simulink model "Simulink_model_171120bslee"  (R2017a)
settings: Solver=ode4  StartTime=0  StopTime=1500  FixedStep=0.01  RelTol=1e-3
model workspace (MAT data in the model file):
  A = 2
  Cd = 0.35
  Jm = 0.05
  Jt = 0.00226
  Jw = 0.905
  Ki = 0.083
  Kp = 0.24
  Nf = 4
  Ni = 2.3
  Rt = 0.316
  f = 0.01
  g = 9.81
  m = 1800
  rho = 1.166
  tout = [0 1 2 3 4 5 6 7 8 9 10 11 ... (51 elements, 51x1)]
  xxx = [0 1 2 3 4 5 6 7 8 9 10 11 ... (15447 elements, 1x15447)]
  yyy = [259 259 259 259 259 259 259 259 259 259 259 259 ... (15447 elements, 1x15447)]
libraries: simulink x1
(part 2 of 2)

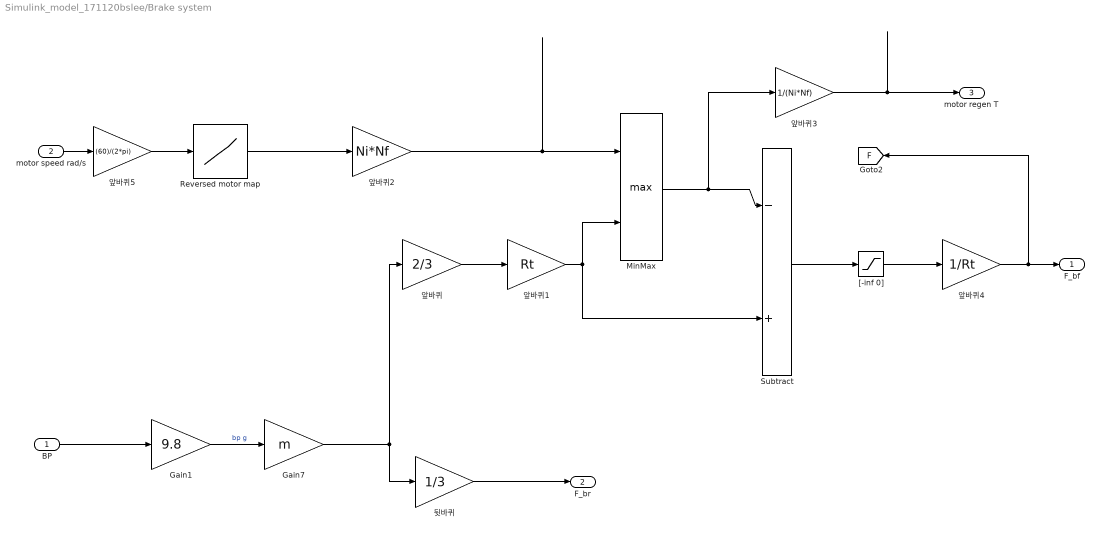
== system Simulink_model_171120bslee/Brake system ==
  BP : Inport
  motor speed rad/s : Inport  Port=2
  Gain1 : Gain  Gain=9.8
  Gain7 : Gain  Gain=m
  MinMax : MinMax  Function=max  Inputs=2
  "Reversed motor map " : Lookup_n-D  NumberOfTableDimensions=1  BreakpointsForDimension1=xxx  Table=yyy*(-1)  InternalRulePriority=Speed  RndMeth=Simplest  InputSameDT=on
  Subtract : Sum  Inputs=-+
  "[-inf 0] " : Saturate  UpperLimit=0  LowerLimit=-inf
  뒷바퀴 : Gain  Gain=1/3
  앞바퀴 : Gain  Gain=2/3
  앞바퀴1 : Gain  Gain=Rt
  앞바퀴2 : Gain  Gain=Ni*Nf
  앞바퀴3 : Gain  Gain=1/(Ni*Nf)
  앞바퀴4 : Gain  Gain=1/Rt
  앞바퀴5 : Gain  Gain=(60)/(2*pi)
  F_bf : Outport
  F_br : Outport  Port=2
  motor regen T : Outport  Port=3
  tag scope: F=global
  wires:
  BP/1 -> Gain1/1
  Gain7/1 -> 뒷바퀴/1, 앞바퀴/1
  Gain1/1 -> Gain7/1  "bp g"
  뒷바퀴/1 -> F_br/1
  앞바퀴2/1 -> MinMax/1
  motor speed rad/s/1 -> 앞바퀴5/1
  MinMax/1 -> 앞바퀴3/1, Subtract/1
  앞바퀴3/1 -> motor regen T/1
  Subtract/1 -> "[-inf 0] "/1
  "[-inf 0] "/1 -> 앞바퀴4/1
  앞바퀴4/1 -> F_bf/1, [F]
  앞바퀴/1 -> 앞바퀴1/1
  앞바퀴1/1 -> MinMax/2, Subtract/2
  앞바퀴5/1 -> "Reversed motor map "/1
  "Reversed motor map "/1 -> 앞바퀴2/1

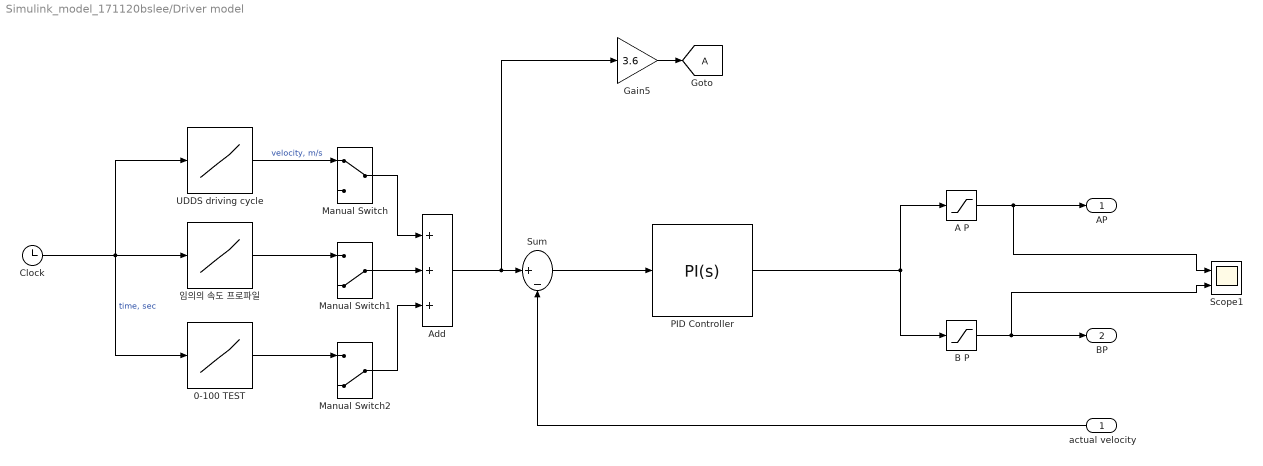
== system Simulink_model_171120bslee/Driver model ==
  actual velocity : Inport
  0-100 TEST : Lookup_n-D  NumberOfTableDimensions=1  BreakpointsForDimension1=[0 0.1 10000]  Table=[0.01 270.778 270.778]  InternalRulePriority=Speed  RndMeth=Simplest  InputSameDT=on
  A P : Saturate  UpperLimit=1  LowerLimit=0
  Add : Sum  Inputs=+++
  "B P " : Saturate  UpperLimit=0  LowerLimit=-1
  Clock : Clock
      settings: Decimation=1000
  Gain5 : Gain  Gain=3.6
  Manual Switch : ManualSwitch
  Manual Switch1 : ManualSwitch  CurrentSetting=0
  Manual Switch2 : ManualSwitch  CurrentSetting=0
  PID Controller : simulink/Continuous/PID Controller  Controller=PI  TimeDomain=Continuous-time  SampleTime=-1  IntegratorMethod=Forward Euler  FilterMethod=Forward Euler  Form=Parallel  UseFilter=on  ControllerParametersSource=internal  P=0.24  I=0.8  D=0  N=100  InitialConditionSource=internal  InitialConditionForIntegrator=0  InitialConditionForFilter=0  ExternalReset=none  LimitOutput=off  UpperSaturationLimit=inf  LowerSaturationLimit=-inf  LinearizeAsGain=on  AntiWindupMode=none  Kb=1  TrackingMode=off  Kt=1  PParamMin=[]  PParamMax=[]  IParamMin=[]  IParamMax=[]  DParamMin=[]  DParamMax=[]  NParamMin=[]  NParamMax=[]  KbParamMin=[]  KbParamMax=[]  KtParamMin=[]  KtParamMax=[]  POutMin=[]  POutMax=[]  IOutMin=[]  IOutMax=[]  DOutMin=[]  DOutMax=[]  NOutMin=[]  NOutMax=[]  KbOutMin=[]  KbOutMax=[]  KtOutMin=[]  KtOutMax=[]  IntegratorOutMin=[]  IntegratorOutMax=[]  FilterOutMin=[]  FilterOutMax=[]  SumOutMin=[]  SumOutMax=[]  SumI1OutMin=[]  SumI1OutMax=[]  SumI2OutMin=[]  SumI2OutMax=[]  SumI3OutMin=[]  SumI3OutMax=[]  SumDOutMin=[]  SumDOutMax=[]  SaturationOutMin=[]  SaturationOutMax=[]  IntegratorContinuousStateAttributes=''  IntegratorStateMustResolveToSignalObject=off  IntegratorRTWStateStorageClass=Auto  FilterContinuousStateAttributes=''  FilterStateMustResolveToSignalObject=off  FilterRTWStateStorageClass=Auto  DifferentiatorICPrevScaledInput=0  DifferentiatorOutMin=[]  DifferentiatorOutMax=[]  InitialConditionSetting=State (most efficient)
  Scope1 : Scope  NumInputPorts=2
  Sum : Sum  Inputs=|+-
  UDDS driving cycle : Lookup  InputValues=|  Table=|
      InputValues=|
      | [0	1	2	3	4	5	6	7	8	9	10	11	12	13	14	15	16	17	18	19	20	21	22	23	24	25	26	27	28	29	30	31	32	33	34	35	36	37	38	39	40	41	42	43	44	45	46	47	48	49	50	51	52	53	54	55	56	57	58	59	60	61	62	63	64	65	66	67	68	69	70	71	72	73	74	75	76	77	78	79	80	81	82	83	84	85	86	87	88	89	90	91	92	93	94	95	96	97	98	99	100	101	102	103	104	105	106	107	108	109	110	111	112	113	114	115	116	117	118	119	120	121	122	123	124	125	126	127	128	129	130	131	132	133	134	135	136	137	138	139	140	141	142	143	144	145	146	147	148	149	150	151	152	153	154	155	156	157	158	159	160	161	162	163	164	165	166	167	168	169	170	171	172	173	174	175	176	177	178	179	180	181	182	183	184	185	186	187	188	189	190	191	192	193	194	195	196	197	198	199	200	201	202	203	204	205	206	207	208	209	210	211	212	213	214	215	216	217	218	219	220	221	222	223	224	225	226	227	228	229	230	231	232	233	234	235	236	237	238	239	240	241	242	243	244	245	246	247	248	249	250	251	252	253	254	255	256	257	258	259	260	261	262	263	264	265	266	267	268	269	270	271	272	273	274	275	276	277	278	279	280	281	282	283	284	285	286	287	288	289	290	291	292	293	294	295	296	297	298	299	300	301	302	303	304	305	306	307	308	309	310	311	312	313	314	315	316	317	318	319	320	321	322	323	324	325	326	327	328	329	330	331	332	333	334	335	336	337	338	339	340	341	342	343	344	345	346	347	348	349	350	351	352	353	354	355	356	357	358	359	360	361	362	363	364	365	366	367	368	369	370	371	372	373	374	375	376	377	378	379	380	381	382	383	384	385	386	387	388	389	390	391	392	393	394	395	396	397	398	399	400	401	402	403	404	405	406	407	408	409	410	411	412	413	414	415	416	417	418	419	420	421	422	423	424	425	426	427	428	429	430	431	432	433	434	435	436	437	438	439	440	441	442	443	444	445	446	447	448	449	450	451	452	453	454	455	456	457	458	459	460	461	462	463	464	465	466	467	468	469	470	471	472	473	474	475	476	477	478	479	480	481	482	483	484	485	486	487	488	489	490	491	492	493	494	495	496	497	498	499	500	501	502	503	504	505	506	507	508	509	510	511	512	513	514	515	516	517	518	519	520	521	522	523	524	525	526	527	528	529	530	531	532	533	534	535	536	537	538	539	540	541	542	543	544	545	546	547	548	549	550	551	552	553	554	555	556	557	558	559	560	561	562	563	564	565	566	567	568	569	570	571	572	573	574	575	576	577	578	579	580	581	582	583	584	585	586	587	588	589	590	591	592	593	594	595	596	597	598	599	600	601	602	603	604	605	606	607	608	609	610	611	612	613	614	615	616	617	618	619	620	621	622	623	624	625	626	627	628	629	630	631	632	633	634	635	636	637	638	639	640	641	642	643	644	645	646	647	648	649	650	651	652	653	654	655	656	657	658	659	660	661	662	663	664	665	666	667	668	669	670	671	672	673	674	675	676	677	678	679	680	681	682	683	684	685	686	687	688	689	690	691	692	693	694	695	696	697	698	699	700	701	702	703	704	705	706	707	708	709	710	711	712	713	714	715	716	717	718	719	720	721	722	723	724	725	726	727	728	729	730	731	732	733	734	735	736	737	738	739	740	741	742	743	744	745	746	747	748	749	750	751	752	753	754	755	756	757	758	759	760	761	762	763	764	765	766	767	768	769	770	771	772	773	774	775	776	777	778	779	780	781	782	783	784	785	786	787	788	789	790	791	792	793	794	795	796	797	798	799	800	801	802	803	804	805	806	807	808	809	810	811	812	813	814	815	816	817	818	819	820	821	822	823	824	825	826	827	828	829	830	831	832	833	834	835	836	837	838	839	840	841	842	843	844	845	846	847	848	849	850	851	852	853	854	855	856	857	858	859	860	861	862	863	864	865	866	867	868	869	870	871	872	873	874	875	876	877	878	879	880	881	882	883	884	885	886	887	888	889	890	891	892	893	894	895	896	897	898	899	900	901	902	903	904	905	906	907	908	909	910	911	912	913	914	915	916	917	918	919	920	921	922	923	924	925	926	927	928	929	930	931	932	933	934	935	936	937	938	939	940	941	942	943	944	945	946	947	948	949	950	951	952	953	954	955	956	957	958	959	960	961	962	963	964	965	966	967	968	969	970	971	972	973	974	975	976	977	978	979	980	981	982	983	984	985	986	987	988	989	990	991	992	993	994	995	996	997	998	999	1000	1001	1002	1003	1004	1005	1006	1007	1008	1009	1010	1011	1012	1013	1014	1015	1016	1017	1018	1019	1020	1021	1022	1023	1024	1025	1026	1027	1028	1029	1030	1031	1032	1033	1034	1035	1036	1037	1038	1039	1040	1041	1042	1043	1044	1045	1046	1047	1048	1049	1050	1051	1052	1053	1054	1055	1056	1057	1058	1059	1060	1061	1062	1063	1064	1065	1066	1067	1068	1069	1070	1071	1072	1073	1074	1075	1076	1077	1078	1079	1080	1081	1082	1083	1084	1085	1086	1087	1088	1089	1090	1091	1092	1093	1094	1095	1096	1097	1098	1099	1100	1101	1102	1103	1104	1105	1106	1107	1108	1109	1110	1111	1112	1113	1114	1115	1116	1117	1118	1119	1120	1121	1122	1123	1124	1125	1126	1127	1128	1129	1130	1131	1132	1133	1134	1135	1136	1137	1138	1139	1140	1141	1142	1143	1144	1145	1146	1147	1148	1149	1150	1151	1152	1153	1154	1155	1156	1157	1158	1159	1160	1161	1162	1163	1164	1165	1166	1167	1168	1169	1170	1171	1172	1173	1174	1175	1176	1177	1178	1179	1180	1181	1182	1183	1184	1185	1186	1187	1188	1189	1190	1191	1192	1193	1194	1195	1196	1197	1198	1199	1200	1201	1202	1203	1204	1205	1206	1207	1208	1209	1210	1211	1212	1213	1214	1215	1216	1217	1218	1219	1220	1221	1222	1223	1224	1225	1226	1227	1228	1229	1230	1231	1232	1233	1234	1235	1236	1237	1238	1239	1240	1241	1242	1243	1244	1245	1246	1247	1248	1249	1250	1251	1252	1253	1254	1255	1256	1257	1258	1259	1260	1261	1262	1263	1264	1265	1266	1267	1268	1269	1270	1271	1272	1273	1274	1275	1276	1277	1278	1279	1280	1281	1282	1283	1284	1285	1286	1287	1288	1289	1290	1291	1292	1293	1294	1295	1296	1297	1298	1299	1300	1301	1302	1303	1304	1305	1306	1307	1308	1309	1310	1311	1312	1313	1314	1315	1316	1317	1318	1319	1320	1321	1322	1323	1324	1325	1326	1327	1328	1329	1330	1331	1332	1333	1334	1335	1336	1337	1338	1339	1340	1341	1342	1343	1344	1345	1346	1347	1348	1349	1350	1351	1352	1353	1354	1355	1356	1357	1358	1359	1360	1361	1362	1363	1364	1365	1366	1367	1368	1369
      | ]
      Table=|
      | [0
      | 0
      | 0
      | 0
      | 0
      | 0
      | 0
      | 0
      | 0
      | 0
      | 0
      | 0
      | 0
      | 0
      | 0
      | 0
      | 0
      | 0
      | 0
      | 0
      | 0
      | 1.34112000000000
      | 2.63753600000000
      | 3.84454400000000
      | 5.14096000000000
      | 6.39267200000000
      | 7.55497600000000
      | 7.73379200000000
      | 8.09142400000000
      | 9.25372800000000
      | 9.70076800000000
      | 10.0136960000000
      | 10.0584000000000
      | 9.87958400000000
      | 9.61136000000000
      | 9.34313600000000
      | 9.11961600000000
      | 8.85139200000000
      | 7.59968000000000
      | 6.66089600000000
      | 6.66089600000000
      | 6.79500800000000
      | 6.92912000000000
      | 7.15264000000000
      | 7.64438400000000
      | 8.53846400000000
      | 9.43254400000000
      | 10.1478080000000
      | 10.2372160000000
      | 10.1478080000000
      | 10.1031040000000
      | 9.52195200000000
      | 8.49376000000000
      | 7.64438400000000
      | 7.06323200000000
      | 7.06323200000000
      | 7.91260800000000
      | 8.85139200000000
      | 9.65606400000000
      | 10.3713280000000
      | 10.8183680000000
      | 10.9971840000000
      | 11.1312960000000
      | 11.1760000000000
      | 10.9971840000000
      | 10.9524800000000
      | 11.0418880000000
      | 11.0865920000000
      | 11.0418880000000
      | 10.9971840000000
      | 10.9971840000000
      | 11.2207040000000
      | 11.4442240000000
      | 11.4889280000000
      | 11.3548160000000
      | 11.1312960000000
      | 11.1760000000000
      | 11.3548160000000
      | 11.6230400000000
      | 11.6230400000000
      | 11.4889280000000
      | 11.6677440000000
      | 11.9359680000000
      | 12.2936000000000
      | 12.7853440000000
      | 13.0982720000000
      | 13.3217920000000
      | 13.4559040000000
      | 13.5900160000000
      | 13.7241280000000
      | 13.7241280000000
      | 13.6347200000000
      | 13.5900160000000
      | 13.5453120000000
      | 13.5900160000000
      | 13.7688320000000
      | 13.5900160000000
      | 13.3664960000000
      | 13.1876800000000
      | 13.3217920000000
      | 13.5453120000000
      | 13.7241280000000
      | 13.8135360000000
      | 13.8582400000000
      | 13.8135360000000
      | 13.5900160000000
      | 13.3217920000000
      | 13.3664960000000
      | 13.5006080000000
      | 13.7241280000000
      | 13.9476480000000
      | 14.2158720000000
      | 14.3946880000000
      | 14.4840960000000
      | 14.3946880000000
      | 14.1711680000000
      | 12.7853440000000
      | 11.3101120000000
      | 9.83488000000000
      | 8.35964800000000
      | 6.88441600000000
      | 5.40918400000000
      | 3.93395200000000
      | 2.45872000000000
      | 0.983488000000000
      | 0
      | 0
      | 0
      | 0
      | 0
      | 0
      | 0
      | 0
      | 0
      | 0
      | 0
      | 0
      | 0
      | 0
      | 0
      | 0
      | 0
      | 0
      | 0
      | 0
      | 0
      | 0
      | 0
      | 0
      | 0
      | 0
      | 0
      | 0
      | 0
      | 0
      | 0
      | 0
      | 0
      | 0
      | 0
      | 0
      | 0
      | 0
      | 0
      | 1.47523200000000
      | 2.95046400000000
      | 4.42569600000000
      | 5.90092800000000
      | 7.37616000000000
      | 8.85139200000000
      | 9.92428800000000
      | 10.8630720000000
      | 11.5336320000000
      | 11.8018560000000
      | 11.4889280000000
      | 11.2207040000000
      | 11.0418880000000
      | 11.1760000000000
      | 11.2654080000000
      | 11.3548160000000
      | 11.5336320000000
      | 12.1594880000000
      | 11.8465600000000
      | 10.7289600000000
      | 10.1478080000000
      | 8.67257600000000
      | 7.91260800000000
      | 7.68908800000000
      | 8.09142400000000
      | 8.31494400000000
      | 8.94080000000000
      | 9.92428800000000
      | 10.9524800000000
      | 12.2041920000000
      | 13.6347200000000
      | 14.9758400000000
      | 16.1828480000000
      | 16.6745920000000
      | 17.5686720000000
      | 18.1051200000000
      | 18.8203840000000
      | 19.4462400000000
      | 20.1615040000000
      | 20.5638400000000
      | 20.9214720000000
      | 21.2344000000000
      | 21.2344000000000
      | 21.1449920000000
      | 21.1002880000000
      | 21.0108800000000
      | 21.0108800000000
      | 21.0108800000000
      | 21.0108800000000
      | 21.0108800000000
      | 21.1002880000000
      | 21.1896960000000
      | 21.4132160000000
      | 21.6814400000000
      | 21.9496640000000
      | 22.1284800000000
      | 22.3520000000000
      | 22.6202240000000
      | 22.7990400000000
      | 23.0225600000000
      | 23.3354880000000
      | 23.7825280000000
      | 24.1848640000000
      | 24.4083840000000
      | 24.5424960000000
      | 24.5872000000000
      | 24.5424960000000
      | 24.4083840000000
      | 24.4083840000000
      | 24.4977920000000
      | 24.6319040000000
      | 24.8107200000000
      | 24.9001280000000
      | 25.0789440000000
      | 25.1683520000000
      | 25.3024640000000
      | 25.3471680000000
      | 25.3471680000000
      | 25.2577600000000
      | 25.2577600000000
      | 25.2577600000000
      | 25.2577600000000
      | 25.2577600000000
      | 25.2577600000000
      | 25.2130560000000
      | 25.0789440000000
      | 24.9448320000000
      | 24.6319040000000
      | 24.4083840000000
      | 24.2295680000000
      | 24.1401600000000
      | 24.0060480000000
      | 23.9613440000000
      | 24.0954560000000
      | 24.1401600000000
      | 24.1848640000000
      | 24.1848640000000
      | 24.0507520000000
      | 23.8719360000000
      | 23.6931200000000
      | 23.5143040000000
      | 23.2907840000000
      | 23.4248960000000
      | 23.2460800000000
      | 23.2013760000000
      | 23.1119680000000
      | 23.0225600000000
      | 23.0672640000000
      | 23.1566720000000
      | 23.2907840000000
      | 23.4696000000000
      | 23.6931200000000
      | 23.9166400000000
      | 24.1401600000000
      | 24.5424960000000
      | 24.7660160000000
      | 24.8554240000000
      | 25.0342400000000
      | 25.0342400000000
      | 24.9448320000000
      | 24.6766080000000
      | 24.3636800000000
      | 23.9613440000000
      | 23.4696000000000
      | 23.0225600000000
      | 23.0225600000000
      | 23.0225600000000
      | 22.8437440000000
      | 22.3967040000000
      | 22.3520000000000
      | 22.3967040000000
      | 22.3520000000000
      | 22.1731840000000
      | 22.1284800000000
      | 22.1284800000000
      | 22.1284800000000
      | 21.9496640000000
      | 21.7261440000000
      | 21.5026240000000
      | 21.1002880000000
      | 20.6085440000000
      | 20.1168000000000
      | 19.5803520000000
      | 19.0439040000000
      | 18.5521600000000
      | 18.0157120000000
      | 17.2110400000000
      | 16.5404800000000
      | 15.7358080000000
      | 15.1099520000000
      | 14.5288000000000
      | 14.0817600000000
      | 13.6794240000000
      | 13.6347200000000
      | 13.4112000000000
      | 12.9641600000000
      | 12.2936000000000
      | 11.0865920000000
      | 9.61136000000000
      | 8.98550400000000
      | 8.53846400000000
      | 8.27024000000000
      | 7.59968000000000
      | 6.92912000000000
      | 5.58800000000000
      | 4.82803200000000
      | 3.57632000000000
      | 2.10108800000000
      | 0.625856000000000
      | 0
      | 0
      | 0
      | 0
      | 0
      | 0
      | 0
      | 0
      | 0
      | 0
      | 0
      | 0
      | 0
      | 0
      | 0.447040000000000
      | 1.92227200000000
      | 3.39750400000000
      | 4.87273600000000
      | 6.34796800000000
      | 7.73379200000000
      | 8.94080000000000
      | 10.0584000000000
      | 10.5948480000000
      | 11.2654080000000
      | 11.8912640000000
      | 12.5618240000000
      | 13.4112000000000
      | 13.7688320000000
      | 14.1264640000000
      | 14.3499840000000
      | 14.6629120000000
      | 15.0205440000000
      | 15.4228800000000
      | 15.4675840000000
      | 15.6016960000000
      | 15.5569920000000
      | 15.4228800000000
      | 15.5122880000000
      | 15.8699200000000
      | 16.0934400000000
      | 16.0934400000000
      | 16.0934400000000
      | 16.0934400000000
      | 16.0934400000000
      | 16.0934400000000
      | 16.1381440000000
      | 16.2722560000000
      | 16.3169600000000
      | 16.2722560000000
      | 16.0934400000000
      | 15.6911040000000
      | 15.2440640000000
      | 14.9758400000000
      | 14.0370560000000
      | 12.9641600000000
      | 11.4889280000000
      | 10.2819200000000
      | 9.07491200000000
      | 7.82320000000000
      | 6.48208000000000
      | 5.36448000000000
      | 3.88924800000000
      | 2.41401600000000
      | 0.938784000000000
      | 0
      | 0
      | 0
      | 0
      | 0
      | 0
      | 1.16230400000000
      | 2.63753600000000
      | 4.11276800000000
      | 5.58800000000000
      | 7.06323200000000
      | 8.53846400000000
      | 10.0136960000000
      | 11.1760000000000
      | 11.4442240000000
      | 12.2936000000000
      | 12.9641600000000
      | 13.4112000000000
      | 13.4559040000000
      | 13.4112000000000
      | 13.2770880000000
      | 13.0982720000000
      | 12.8747520000000
      | 12.5171200000000
      | 11.1760000000000
      | 9.70076800000000
      | 8.22553600000000
      | 6.75030400000000
      | 5.27507200000000
      | 3.79984000000000
      | 2.32460800000000
      | 0.849376000000000
      | 0
      | 0
      | 0
      | 0
      | 0
      | 0
      | 0
      | 0
      | 0
      | 0
      | 0
      | 0
      | 0
      | 0
      | 0
      | 0
      | 0
      | 0
      | 0
      | 1.47523200000000
      | 2.95046400000000
      | 4.42569600000000
      | 5.90092800000000
      | 7.37616000000000
      | 8.85139200000000
      | 10.3266240000000
      | 11.8018560000000
      | 12.4277120000000
      | 13.0088640000000
      | 14.0817600000000
      | 14.7523200000000
      | 15.0205440000000
      | 15.5569920000000
      | 15.6911040000000
      | 15.9146240000000
      | 16.1381440000000
      | 16.0934400000000
      | 16.1381440000000
      | 16.1828480000000
      | 16.0934400000000
      | 15.9593280000000
      | 16.0934400000000
      | 16.0934400000000
      | 15.9146240000000
      | 15.8699200000000
      | 15.8252160000000
      | 15.7358080000000
      | 15.7358080000000
      | 15.7358080000000
      | 15.7358080000000
      | 15.7358080000000
      | 15.7358080000000
      | 15.6464000000000
      | 15.6911040000000
      | 15.7358080000000
      | 15.8699200000000
      | 15.7358080000000
      | 15.6464000000000
      | 15.6464000000000
      | 15.6464000000000
      | 15.5569920000000
      | 15.4675840000000
      | 15.4228800000000
      | 14.9758400000000
      | 14.3052800000000
      | 13.4559040000000
      | 12.5171200000000
      | 11.3995200000000
      | 10.0584000000000
      | 8.85139200000000
      | 7.37616000000000
      | 5.90092800000000
      | 4.60451200000000
      | 3.21868800000000
      | 1.78816000000000
      | 0.447040000000000
      | 0
      | 0
      | 0
      | 0
      | 0
      | 0
      | 0.536448000000000
      | 1.56464000000000
      | 2.45872000000000
      | 2.90576000000000
      | 3.79984000000000
      | 4.29158400000000
      | 4.69392000000000
      | 5.31977600000000
      | 6.25856000000000
      | 7.15264000000000
      | 7.91260800000000
      | 8.49376000000000
      | 8.98550400000000
      | 9.38784000000000
      | 9.83488000000000
      | 10.2819200000000
      | 10.6395520000000
      | 10.9524800000000
      | 11.1312960000000
      | 11.1760000000000
      | 11.1760000000000
      | 11.1760000000000
      | 11.1760000000000
      | 11.1760000000000
      | 11.1760000000000
      | 11.4442240000000
      | 11.5336320000000
      | 11.6230400000000
      | 11.4442240000000
      | 11.2654080000000
      | 11.1760000000000
      | 11.1760000000000
      | 11.1760000000000
      | 10.9077760000000
      | 10.3266240000000
      | 8.85139200000000
      | 7.37616000000000
      | 5.90092800000000
      | 4.42569600000000
      | 2.95046400000000
      | 1.47523200000000
      | 0
      | 0
      | 0
      | 0
      | 0
      | 0
      | 0
      | 0
      | 0
      | 0
      | 0
      | 0
      | 0
      | 0
      | 0
      | 0
      | 0
      | 1.47523200000000
      | 2.95046400000000
      | 4.42569600000000
      | 5.81152000000000
      | 6.52678400000000
      | 7.15264000000000
      | 7.59968000000000
      | 7.59968000000000
      | 7.59968000000000
      | 7.82320000000000
      | 7.91260800000000
      | 7.91260800000000
      | 7.82320000000000
      | 7.59968000000000
      | 7.55497600000000
      | 7.42086400000000
      | 7.59968000000000
      | 7.64438400000000
      | 7.59968000000000
      | 7.42086400000000
      | 7.37616000000000
      | 7.37616000000000
      | 7.42086400000000
      | 7.59968000000000
      | 7.86790400000000
      | 8.27024000000000
      | 8.58316800000000
      | 9.03020800000000
      | 9.38784000000000
      | 9.43254400000000
      | 9.47724800000000
      | 9.65606400000000
      | 9.83488000000000
      | 10.0136960000000
      | 10.0584000000000
      | 10.0584000000000
      | 10.0584000000000
      | 10.1478080000000
      | 10.5948480000000
      | 11.2207040000000
      | 11.6230400000000
      | 11.8465600000000
      | 12.0700800000000
      | 11.6677440000000
      | 10.1925120000000
      | 8.71728000000000
      | 7.24204800000000
      | 5.76681600000000
      | 4.29158400000000
      | 2.81635200000000
      | 1.34112000000000
      | 0
      | 0
      | 0
      | 0
      | 0
      | 0
      | 0
      | 0
      | 0
      | 0
      | 0
      | 0
      | 0
      | 0
      | 0
      | 0
      | 0
      | 0
      | 0
      | 0
      | 0
      | 0
      | 0
      | 0
      | 0
      | 0
      | 0.894080000000000
      | 2.01168000000000
      | 3.48691200000000
      | 4.55980800000000
      | 5.58800000000000
      | 6.25856000000000
      | 6.83971200000000
      | 7.82320000000000
      | 8.76198400000000
      | 9.38784000000000
      | 9.92428800000000
      | 10.4160320000000
      | 10.9524800000000
      | 11.3101120000000
      | 11.4442240000000
      | 11.6230400000000
      | 11.6677440000000
      | 11.7124480000000
      | 11.7124480000000
      | 11.8018560000000
      | 11.8465600000000
      | 11.8465600000000
      | 11.6230400000000
      | 11.3995200000000
      | 10.5501440000000
      | 9.56665600000000
      | 8.27024000000000
      | 7.33145600000000
      | 6.48208000000000
      | 5.18566400000000
      | 3.88924800000000
      | 2.59283200000000
      | 1.56464000000000
      | 0.894080000000000
      | 0
      | 0
      | 0
      | 0
      | 0
      | 0
      | 0
      | 0
      | 0
      | 0
      | 0
      | 0
      | 0
      | 0
      | 0.625856000000000
      | 1.47523200000000
      | 1.96697600000000
      | 2.90576000000000
      | 4.11276800000000
      | 5.05155200000000
      | 6.03504000000000
      | 6.52678400000000
      | 7.33145600000000
      | 7.46556800000000
      | 7.37616000000000
      | 7.37616000000000
      | 8.13612800000000
      | 8.58316800000000
      | 8.98550400000000
      | 9.61136000000000
      | 10.0584000000000
      | 10.0584000000000
      | 9.87958400000000
      | 10.1478080000000
      | 10.4160320000000
      | 10.5054400000000
      | 10.0584000000000
      | 9.65606400000000
      | 9.16432000000000
      | 8.04672000000000
      | 6.70560000000000
      | 5.36448000000000
      | 4.02336000000000
      | 2.77164800000000
      | 2.01168000000000
      | 1.34112000000000
      | 0.938784000000000
      | 0.223520000000000
      | 0.223520000000000
      | 1.43052800000000
      | 2.90576000000000
      | 4.29158400000000
      | 5.58800000000000
      | 6.25856000000000
      | 7.15264000000000
      | 8.04672000000000
      | 8.76198400000000
      | 9.61136000000000
      | 10.3266240000000
      | 10.9524800000000
      | 11.3995200000000
      | 11.8465600000000
      | 12.1147840000000
      | 12.3383040000000
      | 12.4724160000000
      | 12.6512320000000
      | 12.7853440000000
      | 12.7853440000000
      | 12.6512320000000
      | 12.6065280000000
      | 12.5171200000000
      | 12.2936000000000
      | 11.9806720000000
      | 11.3995200000000
      | 10.5054400000000
      | 9.61136000000000
      | 8.49376000000000
      | 7.37616000000000
      | 6.66089600000000
      | 5.58800000000000
      | 4.20217600000000
      | 2.77164800000000
      | 1.34112000000000
      | 0.670560000000000
      | 0.670560000000000
      | 0.223520000000000
      | 0
      | 1.34112000000000
      | 2.81635200000000
      | 4.29158400000000
      | 5.76681600000000
      | 7.06323200000000
      | 7.82320000000000
      | 8.22553600000000
      | 8.71728000000000
      | 9.25372800000000
      | 9.83488000000000
      | 10.3713280000000
      | 11.1760000000000
      | 11.8465600000000
      | 12.2936000000000
      | 12.5171200000000
      | 12.6512320000000
      | 12.9194560000000
      | 12.9194560000000
      | 12.9194560000000
      | 12.8747520000000
      | 12.7406400000000
      | 12.6512320000000
      | 12.6512320000000
      | 12.6512320000000
      | 12.6065280000000
      | 12.3383040000000
      | 12.2936000000000
      | 12.2936000000000
      | 12.2936000000000
      | 12.2936000000000
      | 12.2936000000000
      | 12.2936000000000
      | 12.3383040000000
      | 12.5171200000000
      | 12.7406400000000
      | 13.4112000000000
      | 13.8582400000000
      | 14.3052800000000
      | 14.7523200000000
      | 14.7523200000000
      | 15.0205440000000
      | 15.1993600000000
      | 15.3334720000000
      | 15.2887680000000
      | 15.1993600000000
      | 15.1993600000000
      | 15.1546560000000
      | 15.0205440000000
      | 14.7970240000000
      | 14.7523200000000
      | 14.5288000000000
      | 14.3052800000000
      | 14.2605760000000
      | 14.1264640000000
      | 14.0817600000000
      | 13.6794240000000
      | 13.4112000000000
      | 13.3664960000000
      | 13.3664960000000
      | 13.3664960000000
      | 13.3664960000000
      | 13.2323840000000
      | 13.1876800000000
      | 13.1876800000000
      | 13.0982720000000
      | 12.9194560000000
      | 12.6065280000000
      | 12.3830080000000
      | 12.0700800000000
      | 11.3995200000000
      | 10.5948480000000
      | 9.83488000000000
      | 9.16432000000000
      | 8.58316800000000
      | 8.58316800000000
      | 8.98550400000000
      | 9.34313600000000
      | 9.56665600000000
      | 9.83488000000000
      | 10.1031040000000
      | 10.3713280000000
      | 10.7289600000000
      | 11.1760000000000
      | 11.6230400000000
      | 11.8912640000000
      | 11.8912640000000
      | 11.9806720000000
      | 12.0700800000000
      | 12.1594880000000
      | 12.4277120000000
      | 12.5618240000000
      | 12.8747520000000
      | 12.9194560000000
      | 12.9641600000000
      | 13.0088640000000
      | 12.9641600000000
      | 12.5618240000000
      | 12.2936000000000
      | 12.0700800000000
      | 11.5336320000000
      | 11.1760000000000
      | 10.9524800000000
      | 11.0865920000000
      | 11.2207040000000
      | 11.3995200000000
      | 11.4889280000000
      | 11.7124480000000
      | 12.0253760000000
      | 12.2936000000000
      | 12.4277120000000
      | 12.6959360000000
      | 12.9641600000000
      | 13.0535680000000
      | 13.0088640000000
      | 12.9641600000000
      | 12.9194560000000
      | 12.7406400000000
      | 12.5618240000000
      | 12.5171200000000
      | 12.5171200000000
      | 12.3383040000000
      | 12.1594880000000
      | 11.8912640000000
      | 12.0700800000000
      | 12.2936000000000
      | 12.4277120000000
      | 12.5171200000000
      | 12.4277120000000
      | 12.5171200000000
      | 12.5171200000000
      | 12.5171200000000
      | 12.3830080000000
      | 12.2488960000000
      | 12.0253760000000
      | 11.8912640000000
      | 11.8465600000000
      | 11.8465600000000
      | 11.8465600000000
      | 11.7571520000000
      | 11.7124480000000
      | 11.7124480000000
      | 11.5783360000000
      | 11.4442240000000
      | 11.4442240000000
      | 11.5783360000000
      | 11.5336320000000
      | 11.3995200000000
      | 10.9971840000000
      | 10.5054400000000
      | 9.92428800000000
      | 9.65606400000000
      | 9.65606400000000
      | 9.70076800000000
      | 10.1031040000000
      | 10.4607360000000
      | 10.7289600000000
      | 10.8183680000000
      | 10.9077760000000
      | 11.1312960000000
      | 11.2207040000000
      | 11.2654080000000
      | 11.3101120000000
      | 11.3995200000000
      | 11.2654080000000
      | 11.1760000000000
      | 11.1760000000000
      | 11.1760000000000
      | 11.0418880000000
      | 10.9524800000000
      | 10.8630720000000
      | 10.8630720000000
      | 10.9524800000000
      | 11.1760000000000
      | 11.1760000000000
      | 10.9971840000000
      | 10.9971840000000
      | 10.7736640000000
      | 10.9524800000000
      | 11.2207040000000
      | 11.4442240000000
      | 11.2207040000000
      | 10.7289600000000
      | 9.83488000000000
      | 8.98550400000000
      | 7.55497600000000
      | 6.07974400000000
      | 4.60451200000000
      | 3.12928000000000
      | 1.65404800000000
      | 0.178816000000000
      | 0
      | 0
      | 0
      | 0.894080000000000
      | 2.36931200000000
      | 3.84454400000000
      | 5.31977600000000
      | 6.79500800000000
      | 7.82320000000000
      | 8.31494400000000
      | 8.94080000000000
      | 9.43254400000000
      | 9.83488000000000
      | 10.2819200000000
      | 10.9524800000000
      | 11.7571520000000
      | 12.2936000000000
      | 12.5618240000000
      | 12.6959360000000
      | 12.7406400000000
      | 12.7406400000000
      | 12.7406400000000
      | 12.3830080000000
      | 12.2936000000000
      | 12.1594880000000
      | 11.9806720000000
      | 11.8465600000000
      | 11.6230400000000
      | 11.4889280000000
      | 11.2654080000000
      | 10.7289600000000
      | 9.83488000000000
      | 9.61136000000000
      | 9.61136000000000
      | 9.74547200000000
      | 10.0584000000000
      | 10.2819200000000
      | 10.1925120000000
      | 10.1925120000000
      | 10.2819200000000
      | 10.1478080000000
      | 10.1478080000000
      | 10.1478080000000
      | 10.5054400000000
      | 10.7289600000000
      | 10.9971840000000
      | 11.0865920000000
      | 11.2207040000000
      | 11.3995200000000
      | 11.4442240000000
      | 11.3995200000000
      | 11.1760000000000
      | 10.7736640000000
      | 10.5948480000000
      | 10.3713280000000
      | 10.2372160000000
      | 10.0584000000000
      | 9.83488000000000
      | 9.65606400000000
      | 9.16432000000000
      | 7.82320000000000
      | 6.34796800000000
      | 4.87273600000000
      | 3.39750400000000
      | 1.92227200000000
      | 0.447040000000000
      | 0
      | 0
      | 0
      | 0
      | 0
      | 0
      | 0
      | 0
      | 0
      | 0
      | 0
      | 0
      | 0
      | 0
      | 0
      | 0
      | 0
      | 0
      | 0
      | 0
      | 0
      | 0
      | 0
      | 0
      | 0
      | 0
      | 0
      | 0
      | 0
      | 0
      | 0.536448000000000
      | 1.78816000000000
      | 3.26339200000000
      | 4.73862400000000
      | 6.21385600000000
      | 7.59968000000000
      | 8.27024000000000
      | 8.94080000000000
      | 9.74547200000000
      | 10.2819200000000
      | 10.7289600000000
      | 11.0865920000000
      | 11.4442240000000
      | 11.8465600000000
      | 11.9806720000000
      | 12.2488960000000
      | 12.4724160000000
      | 12.6512320000000
      | 12.5171200000000
      | 12.2936000000000
      | 12.0700800000000
      | 12.0700800000000
      | 11.7571520000000
      | 10.9524800000000
      | 10.0584000000000
      | 9.61136000000000
      | 9.20902400000000
      | 8.04672000000000
      | 6.70560000000000
      | 5.49859200000000
      | 4.96214400000000
      | 4.73862400000000
      | 4.47040000000000
      | 4.24688000000000
      | 4.06806400000000
      | 3.88924800000000
      | 3.84454400000000
      | 3.93395200000000
      | 4.02336000000000
      | 3.88924800000000
      | 3.84454400000000
      | 3.57632000000000
      | 3.12928000000000
      | 2.23520000000000
      | 1.87756800000000
      | 1.16230400000000
      | 0.447040000000000
      | 0
      | 0.0447040000000000
      | 0.268224000000000
      | 0.715264000000000
      | 1.60934400000000
      | 3.08457600000000
      | 4.47040000000000
      | 5.72211200000000
      | 6.25856000000000
      | 6.48208000000000
      | 7.15264000000000
      | 8.09142400000000
      | 8.94080000000000
      | 9.38784000000000
      | 9.47724800000000
      | 9.52195200000000
      | 9.56665600000000
      | 9.70076800000000
      | 10.0584000000000
      | 10.2819200000000
      | 10.6395520000000
      | 10.9524800000000
      | 11.1760000000000
      | 11.1312960000000
      | 11.0865920000000
      | 11.1760000000000
      | 11.3548160000000
      | 11.5336320000000
      | 11.6230400000000
      | 11.8018560000000
      | 11.8912640000000
      | 12.0253760000000
      | 12.0700800000000
      | 12.0700800000000
      | 12.0700800000000
      | 12.0253760000000
      | 11.9806720000000
      | 11.9806720000000
      | 11.8465600000000
      | 11.8018560000000
      | 11.6230400000000
      | 11.3995200000000
      | 10.9971840000000
      | 10.5054400000000
      | 9.61136000000000
      | 8.94080000000000
      | 7.82320000000000
      | 7.15264000000000
      | 6.25856000000000
      | 4.78332800000000
      | 3.30809600000000
      | 1.83286400000000
      | 0.357632000000000
      | 0
      | 0
      | 0
      | 0
      | 0
      | 0
      | 0
      | 0
      | 0
      | 0
      | 0
      | 0
      | 0
      | 0
      | 0
      | 0
      | 0.938784000000000
      | 2.41401600000000
      | 3.88924800000000
      | 5.36448000000000
      | 6.83971200000000
      | 8.31494400000000
      | 9.43254400000000
      | 10.2819200000000
      | 10.5054400000000
      | 10.2819200000000
      | 10.0584000000000
      | 8.94080000000000
      | 7.46556800000000
      | 5.99033600000000
      | 4.51510400000000
      | 3.03987200000000
      | 1.56464000000000
      | 0.0894080000000000
      | 0
      | 0
      | 0
      | 0
      | 0
      | 0
      | 0
      | 0
      | 0
      | 0
      | 0.0894080000000000
      | 0.670560000000000
      | 1.56464000000000
      | 2.90576000000000
      | 4.38099200000000
      | 5.36448000000000
      | 5.76681600000000
      | 5.81152000000000
      | 5.63270400000000
      | 5.72211200000000
      | 5.85622400000000
      | 5.85622400000000
      | 6.25856000000000
      | 6.92912000000000
      | 7.59968000000000
      | 8.31494400000000
      | 8.80668800000000
      | 9.38784000000000
      | 9.61136000000000
      | 9.74547200000000
      | 9.74547200000000
      | 9.61136000000000
      | 9.47724800000000
      | 9.61136000000000
      | 9.74547200000000
      | 9.83488000000000
      | 9.79017600000000
      | 9.70076800000000
      | 9.61136000000000
      | 9.61136000000000
      | 9.56665600000000
      | 8.98550400000000
      | 8.71728000000000
      | 8.58316800000000
      | 8.76198400000000
      | 8.85139200000000
      | 8.94080000000000
      | 8.71728000000000
      | 7.82320000000000
      | 6.92912000000000
      | 5.81152000000000
      | 4.47040000000000
      | 3.57632000000000
      | 2.68224000000000
      | 1.78816000000000
      | 1.11760000000000
      | 0.312928000000000
      | 0
      | 0
      | 0
      | 0
      | 0
      | 0
      | 0
      | 0
      | 0.447040000000000
      | 0.447040000000000
      | 0.447040000000000
      | 0.447040000000000
      | 0.447040000000000
      | 0.715264000000000
      | 1.34112000000000
      | 1.78816000000000
      | 2.23520000000000
      | 2.81635200000000
      | 3.57632000000000
      | 4.47040000000000
      | 4.69392000000000
      | 4.24688000000000
      | 3.79984000000000
      | 3.39750400000000
      | 3.93395200000000
      | 4.91744000000000
      | 6.25856000000000
      | 7.59968000000000
      | 8.71728000000000
      | 9.38784000000000
      | 9.74547200000000
      | 9.92428800000000
      | 10.2819200000000
      | 10.5501440000000
      | 10.7736640000000
      | 10.9524800000000
      | 10.9524800000000
      | 10.7289600000000
      | 10.5054400000000
      | 10.5054400000000
      | 10.5054400000000
      | 10.5054400000000
      | 10.5054400000000
      | 10.5054400000000
      | 10.7289600000000
      | 10.7736640000000
      | 10.9524800000000
      | 11.0418880000000
      | 11.1760000000000
      | 11.3548160000000
      | 11.4442240000000
      | 11.4889280000000
      | 11.6230400000000
      | 11.7124480000000
      | 12.0700800000000
      | 12.4277120000000
      | 12.6512320000000
      | 12.9641600000000
      | 13.0088640000000
      | 12.9641600000000
      | 12.5171200000000
      | 11.0418880000000
      | 9.56665600000000
      | 8.09142400000000
      | 6.61619200000000
      | 5.14096000000000
      | 3.66572800000000
      | 2.19049600000000
      | 0.715264000000000
      | 0
      | 0
      | 0
      | 0
      | 0
      | 0
      | 0
      | 0
      | 0
      | 0
      | 0
      | 0
      | 0
      | 0
      | 0
      | 0
      | 0
      | 0
      | 0
      | 0
      | 0
      | 0
      | 0
      | 0
      | 0
      | 0.670560000000000
      | 2.14579200000000
      | 3.62102400000000
      | 5.09625600000000
      | 5.90092800000000
      | 6.75030400000000
      | 7.51027200000000
      | 8.18083200000000
      | 8.71728000000000
      | 9.07491200000000
      | 9.52195200000000
      | 9.79017600000000
      | 9.87958400000000
      | 10.0136960000000
      | 9.83488000000000
      | 9.65606400000000
      | 9.43254400000000
      | 9.16432000000000
      | 8.94080000000000
      | 8.76198400000000
      | 8.27024000000000
      | 7.82320000000000
      | 7.37616000000000
      | 6.92912000000000
      | 6.25856000000000
      | 4.91744000000000
      | 3.57632000000000
      | 2.32460800000000
      | 1.11760000000000
      | 0
      | 0
      | 0
      | ]
  임의의 속도 프로파일 : Lookup_n-D  NumberOfTableDimensions=1  BreakpointsForDimension1=[0 10 100 120 220 620 630 640 650 660 1000 1010 1020 1030 1400 1410 1420 1430 1500]  Table=[0 16.7 16.7 8.4 27.8 27.8 16.7 16.7 8.4 0 0 8.4 16.7 27.8 27.8 16.7 8.4 0 0]  InternalRulePriority=Speed  RndMeth=Simplest  InputSameDT=on
  "AP " : Outport
  BP : Outport  Port=2
  tag scope: A=global
  wires:
  actual velocity/1 -> Sum/2
  Sum/1 -> PID Controller/1
  "B P "/1 -> Scope1/2, BP/1
  Clock/1 -> UDDS driving cycle/1, 임의의 속도 프로파일/1, 0-100 TEST/1  "time, sec"
  UDDS driving cycle/1 -> Manual Switch/1  "velocity, m/s"
  임의의 속도 프로파일/1 -> Manual Switch1/1
  Gain5/1 -> [A]
  0-100 TEST/1 -> Manual Switch2/1
  Manual Switch/1 -> Add/1
  PID Controller/1 -> "B P "/1, A P/1
  Manual Switch2/1 -> Add/3
  Manual Switch1/1 -> Add/2
  Add/1 -> Gain5/1, Sum/1
  A P/1 -> Scope1/1, "AP "/1

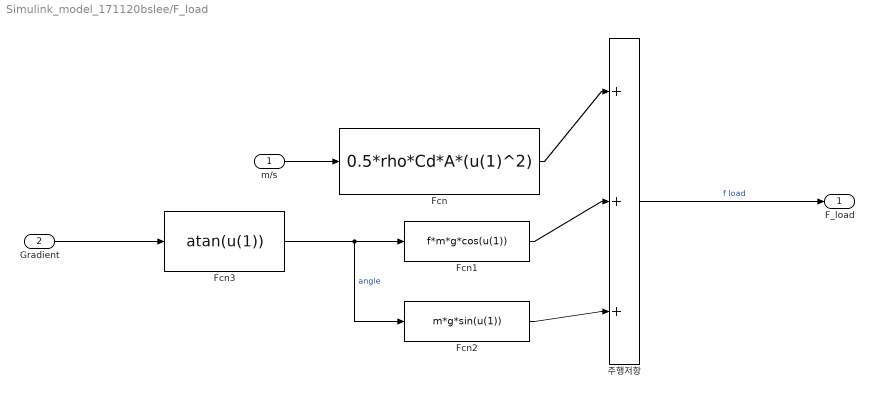
== system Simulink_model_171120bslee/F_load ==
  m/s : Inport
  Gradient : Inport  Port=2
  Fcn : Fcn  Expr=0.5*rho*Cd*A*(u(1)^2)
  Fcn1 : Fcn  Expr=f*m*g*cos(u(1))
  Fcn2 : Fcn  Expr=m*g*sin(u(1))
  Fcn3 : Fcn  Expr=atan(u(1))
  주행저항 : Sum  Inputs=|+++
  F_load : Outport
  wires:
  Fcn1/1 -> 주행저항/2
  Fcn/1 -> 주행저항/1
  Fcn2/1 -> 주행저항/3
  Fcn3/1 -> Fcn2/1, Fcn1/1  "angle"
  주행저항/1 -> F_load/1  "f load"
  Gradient/1 -> Fcn3/1
  m/s/1 -> Fcn/1

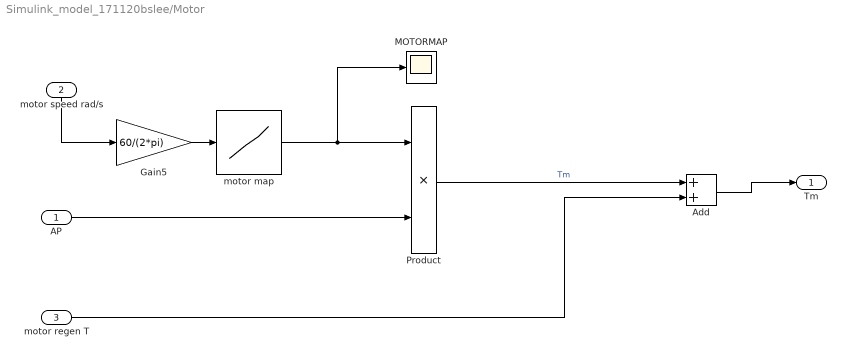
== system Simulink_model_171120bslee/Motor ==
  AP : Inport
  motor speed rad/s : Inport  Port=2
  motor regen T : Inport  Port=3
  Add : Sum
  Gain5 : Gain  Gain=60/(2*pi)
  MOTORMAP : Scope
  Product : Product
  "motor map " : Lookup_n-D  NumberOfTableDimensions=1  BreakpointsForDimension1=xxx  Table=yyy  InternalRulePriority=Speed  RndMeth=Simplest  InputSameDT=on
  Tm : Outport
  wires:
  motor speed rad/s/1 -> Gain5/1
  AP/1 -> Product/2
  Product/1 -> Add/1  "Tm"
  motor regen T/1 -> Add/2
  Add/1 -> Tm/1
  Gain5/1 -> "motor map "/1
  "motor map "/1 -> Product/1, MOTORMAP/1

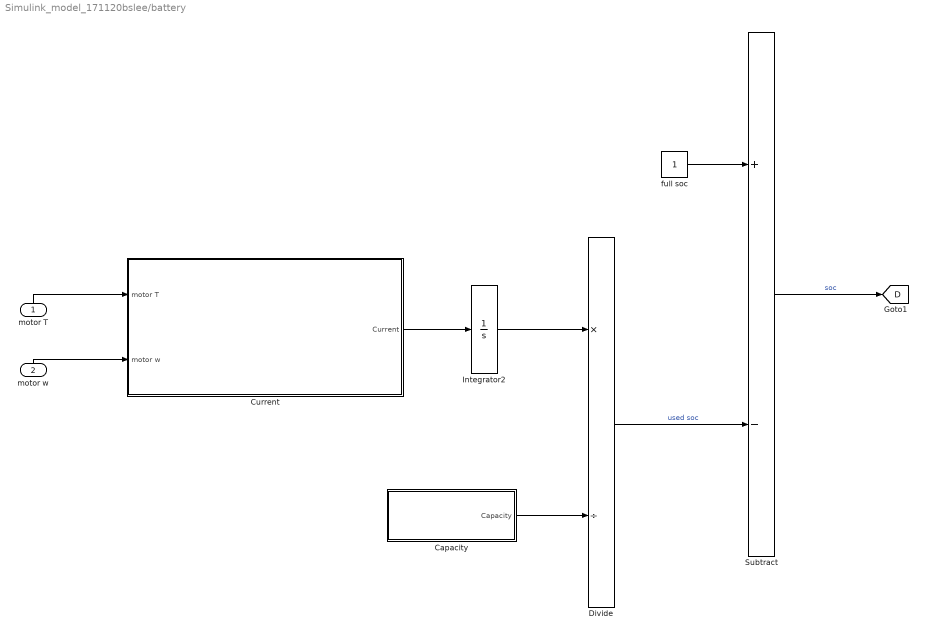
== system Simulink_model_171120bslee/battery ==
  motor T : Inport
  motor w : Inport  Port=2
  Capacity : Subsystem
  Current : Subsystem
  Divide : Product  Inputs=*/
  Integrator2 : Integrator  InitialCondition=0.001
  Subtract : Sum  Inputs=+-
  full soc : Constant
  tag scope: D=global
  wires:
  motor w/1 -> Current/2(motor w)
  motor T/1 -> Current/1(motor T)
  Capacity/1(Capacity) -> Divide/2
  Divide/1 -> Subtract/2  "used soc"
  full soc/1 -> Subtract/1
  Subtract/1 -> [D]  "soc"
  Current/1(Current) -> Integrator2/1
  Integrator2/1 -> Divide/1

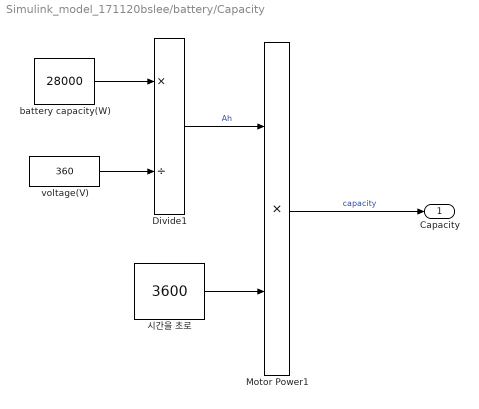
== system Simulink_model_171120bslee/battery/Capacity ==
  Divide1 : Product  Inputs=*/
  Motor Power1 : Product
  battery capacity(W) : Constant  Value=28000
  "voltage(V) " : Constant  Value=360
  시간을 초로 : Constant  Value=3600
  Capacity : Outport
  wires:
  battery capacity(W)/1 -> Divide1/1
  시간을 초로/1 -> Motor Power1/2
  Motor Power1/1 -> Capacity/1  "capacity"
  "voltage(V) "/1 -> Divide1/2
  Divide1/1 -> Motor Power1/1  "Ah"

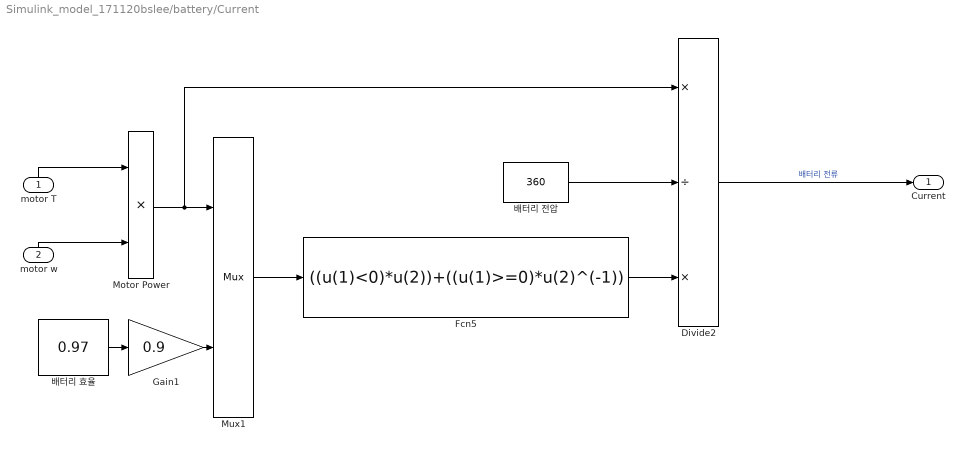
== system Simulink_model_171120bslee/battery/Current ==
  motor T : Inport
  motor w : Inport  Port=2
  Divide2 : Product  Inputs=*/*
  Fcn5 : Fcn  Expr=((u(1)<0)*u(2))+((u(1)>=0)*u(2)^(-1))
  Gain1 : Gain  Gain=0.9
  Motor Power : Product
  Mux1 : Mux  Inputs=2
  "배터리 전압 " : Constant  Value=360
  "배터리 효율 " : Constant  Value=0.97
  Current : Outport
  wires:
  motor w/1 -> Motor Power/2
  motor T/1 -> Motor Power/1
  Fcn5/1 -> Divide2/3
  Divide2/1 -> Current/1  "배터리 전류"
  Motor Power/1 -> Mux1/1, Divide2/1
  "배터리 전압 "/1 -> Divide2/2
  Mux1/1 -> Fcn5/1
  "배터리 효율 "/1 -> Gain1/1
  Gain1/1 -> Mux1/2
